simulink model "mController"  (R2014a)
settings: Solver=ode45  StartTime=0.0  StopTime=ttotal  RelTol=1e-3
values from neighbouring files (symbols this model uses):
  D = Kp*Td    (= 5.058)    [Modeling.m]    (also in model.m = 6.021)
  I = Kp/Ti    (= 2.1053069719)    [Modeling.m]    (also in model.m = 0.403059935166)
  K = Kpp    (= 0.76675)    [Modeling.m]    (also in model.m = 126)
  L = tm    (= 1.55)    [Modeling.m]    (also in model.m = 3.865)
  P = Kp    (= 6.5264516129)    [Modeling.m]    (also in model.m = 3.11565329884)
  T = tau    (= 8.43)    [Modeling.m]    (also in model.m = 10.035)
  ttotal = 200    [Modeling.m]    (also in model.m)
settings Model: Creator=jEdwin  LastModifiedBy=jEdwin

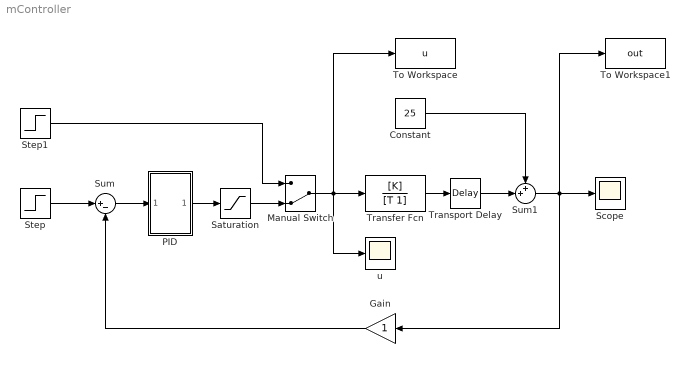
== system mController ==
  Constant : Constant  Value=25  SampleTime=-1
  Gain : Gain  SaturateOnIntegerOverflow=on  OutDataTypeStr=Inherit: Same as input  ParamDataTypeStr=Inherit: Same as input
  Manual Switch : ManualSwitch  CurrentSetting=0
  PID : Subsystem
  Saturation : Saturate  UpperLimit=100  LowerLimit=0
  Scope : Scope
  Step : Step  Time=0  After=30  SampleTime=0.01
  Step1 : Step  Time=ttotal/2  Before=10  After=50  SampleTime=0
  Sum : Sum  Inputs=|+-  SaturateOnIntegerOverflow=on
  Sum1 : Sum  Inputs=++|  SaturateOnIntegerOverflow=on
  To Workspace : ToWorkspace  VariableName=u  SaveFormat=Structure With Time  SampleTime=-1
  To Workspace1 : ToWorkspace  VariableName=out  SaveFormat=Structure With Time  SampleTime=-1
  Transfer Fcn : TransferFcn  Numerator=[K]  Denominator=[T 1]
  Transport Delay : TransportDelay  DelayTime=L
  u : Scope
  wires:
  Step/1 -> Sum/1
  Gain/1 -> Sum/2
  Manual Switch/1 -> To Workspace/1, u/1, Transfer Fcn/1
  PID/1(Out1) -> Saturation/1
  Sum/1 -> PID/1(In1)
  Constant/1 -> Sum1/1
  Saturation/1 -> Manual Switch/2
  Step1/1 -> Manual Switch/1
  Transfer Fcn/1 -> Transport Delay/1
  Transport Delay/1 -> Sum1/2
  Sum1/1 -> To Workspace1/1, Gain/1, Scope/1

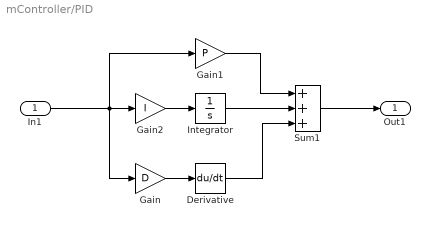
== system mController/PID ==
  In1 : Inport
  Derivative : Derivative
  Gain : Gain  Gain=D  SaturateOnIntegerOverflow=on  OutDataTypeStr=Inherit: Same as input  ParamDataTypeStr=Inherit: Same as input
  Gain1 : Gain  Gain=P  SaturateOnIntegerOverflow=on  OutDataTypeStr=Inherit: Same as input  ParamDataTypeStr=Inherit: Same as input
  Gain2 : Gain  Gain=I  SaturateOnIntegerOverflow=on  OutDataTypeStr=Inherit: Same as input  ParamDataTypeStr=Inherit: Same as input
  Integrator : Integrator
  Sum1 : Sum  Inputs=+++
  Out1 : Outport
  wires:
  Gain1/1 -> Sum1/1
  Derivative/1 -> Sum1/3
  Integrator/1 -> Sum1/2
  In1/1 -> Gain1/1, Gain2/1, Gain/1
  Gain/1 -> Derivative/1
  Sum1/1 -> Out1/1
  Gain2/1 -> Integrator/1
